simulink model "multirateEKFExample"  (R2018a)
settings: Solver=VariableStepAuto  StartTime=0.0  StopTime=t(end)  RelTol=1e-3
values from neighbouring files (symbols this model uses):
  Ts = 0.05    [MultirateNonlinearStateEstimationInSimulinkExample.m]
libraries: simulink x2, sharedTrackingLibrary x1
settings Model: Creator=The MathWorks, Inc.  LastModifiedBy=The MathWorks, Inc.
settings CodeAppCC: StateflowObjectComments=on

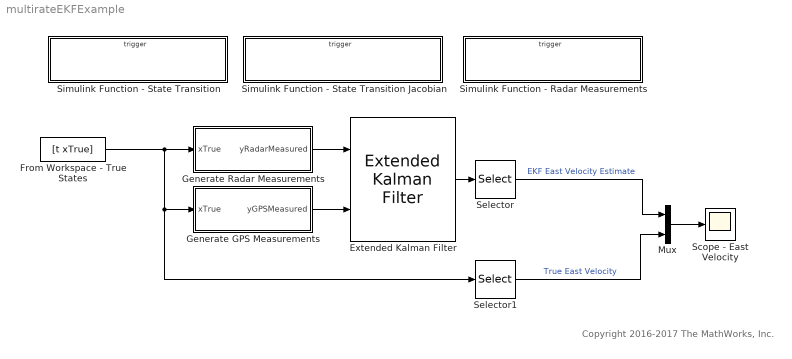
== system multirateEKFExample ==
  note: Copyright 2016-2017 The MathWorks, Inc.
  Extended Kalman Filter : sharedTrackingLibrary/Extended Kalman Filter  StateTransitionFcn=stateTransitionFcn  HasStateTransitionJacobianFcn=on  StateTransitionJacobianFcn=stateTransitionJacobianFcn  HasAdditiveProcessNoise=Nonadditive  ProcessNoise=[0.2 0; 0 0.2]  HasTimeVaryingProcessNoise=off  HasStateTransitionFcnExtraArgument=0  InitialState=[100; 100; 0; 0]  InitialStateCovariance=10  MeasurementFcn1=radarMeasurementFcn  HasMeasurementJacobianFcn1=off  HasMeasurementEnablePort1=off  HasAdditiveMeasurementNoise1=Nonadditive  MeasurementNoise1=[0.0025 0; 0 0.0025]  HasTimeVaryingMeasurementNoise1=off  HasMeasurementFcnExtraArgument1=0  MeasurementFcn2=gpsMeasurementFcn  HasMeasurementJacobianFcn2=off  HasMeasurementEnablePort2=off  HasAdditiveMeasurementNoise2=Additive  MeasurementNoise2=[100 0; 0 100]  HasTimeVaryingMeasurementNoise2=off  HasMeasurementFcnExtraArgument2=0  MeasurementFcn3=myMeasurementFcn  HasMeasurementJacobianFcn3=off  HasMeasurementEnablePort3=off  HasAdditiveMeasurementNoise3=Additive  MeasurementNoise3=1  HasTimeVaryingMeasurementNoise3=off  HasMeasurementFcnExtraArgument3=0  MeasurementFcn4=myMeasurementFcn  HasMeasurementJacobianFcn4=off  HasMeasurementEnablePort4=off  HasAdditiveMeasurementNoise4=Additive  MeasurementNoise4=1  HasTimeVaryingMeasurementNoise4=off  HasMeasurementFcnExtraArgument4=0  MeasurementFcn5=myMeasurementFcn  HasMeasurementJacobianFcn5=off  HasMeasurementEnablePort5=off  HasAdditiveMeasurementNoise5=Additive  MeasurementNoise5=1  HasTimeVaryingMeasurementNoise5=off  HasMeasurementFcnExtraArgument5=0  EnableMultirate=on  StateTransitionFcnSampleTime=0.05  MeasurementFcn1SampleTime=0.05  MeasurementFcn2SampleTime=1  MeasurementFcn3SampleTime=-1  MeasurementFcn4SampleTime=-1  MeasurementFcn5SampleTime=-1  UseCurrentEstimator=on  OutputStateCovariance=off  DataType=double  SampleTime=1  NumberOfMeasurements=2
      settings: SourceProductName=Control System Toolbox  SourceProductBaseCode=CT
  From Workspace - True States : FromWorkspace  VariableName=[t xTrue]  SampleTime=0
  Generate GPS Measurements : Subsystem
  Generate Radar Measurements : Subsystem
  Mux : Mux  Inputs=2
  Scope - East Velocity : Scope
  Selector : Selector  InputPortWidth=4  IndexOptions=Index vector (dialog)  Indices=3  OutputSizes=1
  Selector1 : Selector  InputPortWidth=4  IndexOptions=Index vector (dialog)  Indices=3  OutputSizes=1
  Simulink Function - Radar Measurements : Subsystem  TreatAsAtomicUnit=on
  Simulink Function - State Transition : Subsystem  TreatAsAtomicUnit=on
  Simulink Function - State Transition Jacobian : Subsystem  TreatAsAtomicUnit=on
  wires:
  From Workspace - True States/1 -> Selector1/1, Generate GPS Measurements/1(xTrue), Generate Radar Measurements/1(xTrue)
  Generate Radar Measurements/1(yRadarMeasured) -> Extended Kalman Filter/1
  Generate GPS Measurements/1(yGPSMeasured) -> Extended Kalman Filter/2
  Mux/1 -> Scope - East Velocity/1
  Selector1/1 -> Mux/2  "True East Velocity"
  Selector/1 -> Mux/1  "EKF East Velocity Estimate"
  Extended Kalman Filter/1 -> Selector/1

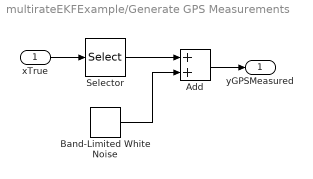
== system multirateEKFExample/Generate GPS Measurements ==
  xTrue : Inport  SampleTime=20*Ts
  Add : Sum
  Band-Limited White Noise : simulink/Sources/Band-Limited White Noise  Cov=50  Ts=20*Ts  seed=[23343;23344]
  Selector : Selector  InputPortWidth=4  IndexOptions=Index vector (dialog)  Indices=[1:2]  OutputSizes=1
  yGPSMeasured : Outport
  wires:
  xTrue/1 -> Selector/1
  Selector/1 -> Add/1
  Add/1 -> yGPSMeasured/1
  Band-Limited White Noise/1 -> Add/2

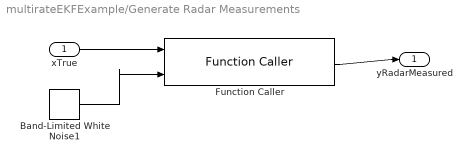
== system multirateEKFExample/Generate Radar Measurements ==
  xTrue : Inport  SampleTime=0.05
  Band-Limited White Noise1 : simulink/Sources/Band-Limited White Noise  Cov=5e-5  Ts=0.05  seed=[23341;23342]
  Function Caller : FunctionCaller  FunctionPrototype=y = radarMeasurementFcn(x,v)  InputArgumentSpecifications=zeros(4,1), zeros(2,1)  OutputArgumentSpecifications=zeros(2,1)
  yRadarMeasured : Outport
  wires:
  Function Caller/1 -> yRadarMeasured/1
  xTrue/1 -> Function Caller/1
  Band-Limited White Noise1/1 -> Function Caller/2

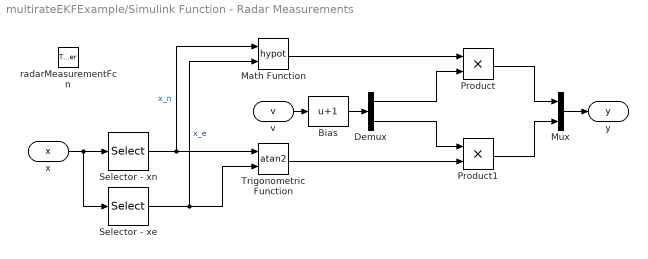
== system multirateEKFExample/Simulink Function - Radar Measurements ==
  radarMeasurementFcn : TriggerPort  TriggerType=function-call  IsSimulinkFunction=on  FunctionName=radarMeasurementFcn  VariantControl=Variant
  Bias : Bias  Bias=1
  Demux : Demux  Outputs=2
  Math Function : Math  Operator=hypot  SaturateOnIntegerOverflow=on
  Mux : Mux  Inputs=2
  Product : Product
  Product1 : Product
  Selector - xe : Selector  InputPortWidth=4  IndexOptions=Index vector (dialog)  Indices=1  OutputSizes=1
  Selector - xn : Selector  InputPortWidth=4  IndexOptions=Index vector (dialog)  Indices=2  OutputSizes=1
  Trigonometric Function : Trigonometry  Operator=atan2
  x : ArgIn  DisableCoverage=on  PortDimensions=4  ArgumentName=x
  v : ArgIn  DisableCoverage=on  Port=2  PortDimensions=2  ArgumentName=v
  y : ArgOut  DisableCoverage=on  PortDimensions=2  ArgumentName=y
  wires:
  Mux/1 -> y/1
  x/1 -> Selector - xe/1, Selector - xn/1
  Selector - xn/1 -> Math Function/1, Trigonometric Function/1  "x_n"
  Selector - xe/1 -> Math Function/2, Trigonometric Function/2  "x_e"
  Trigonometric Function/1 -> Product1/2
  v/1 -> Bias/1
  Math Function/1 -> Product/1
  Product/1 -> Mux/1
  Product1/1 -> Mux/2
  Bias/1 -> Demux/1
  Demux/1 -> Product/2
  Demux/2 -> Product1/1

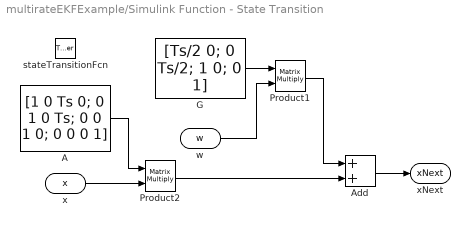
== system multirateEKFExample/Simulink Function - State Transition ==
  stateTransitionFcn : TriggerPort  TriggerType=function-call  IsSimulinkFunction=on  FunctionName=stateTransitionFcn  VariantControl=Variant
  A : Constant  Value=[1 0 Ts 0; 0 1 0 Ts; 0 0 1 0; 0 0 0 1]
  Add : Sum
  G : Constant  Value=[Ts/2 0; 0 Ts/2; 1 0; 0 1]
  Product1 : Product  Multiplication=Matrix(*)
  Product2 : Product  Multiplication=Matrix(*)
  x : ArgIn  DisableCoverage=on  PortDimensions=4  ArgumentName=x
  w : ArgIn  Port=2  PortDimensions=2  ArgumentName=w
  xNext : ArgOut  DisableCoverage=on  PortDimensions=4  ArgumentName=xNext
  wires:
  x/1 -> Product2/2
  A/1 -> Product2/1
  Product2/1 -> Add/2
  G/1 -> Product1/1
  w/1 -> Product1/2
  Product1/1 -> Add/1
  Add/1 -> xNext/1

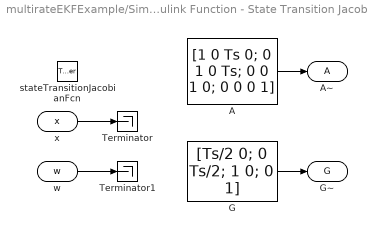
== system multirateEKFExample/Simulink Function - State Transition Jacobian ==
  stateTransitionJacobianFcn : TriggerPort  TriggerType=function-call  IsSimulinkFunction=on  FunctionName=stateTransitionJacobianFcn  VariantControl=Variant
  A : Constant  Value=[1 0 Ts 0; 0 1 0 Ts; 0 0 1 0; 0 0 0 1]
  G : Constant  Value=[Ts/2 0; 0 Ts/2; 1 0; 0 1]
  Terminator : Terminator
  Terminator1 : Terminator
  x : ArgIn  DisableCoverage=on  PortDimensions=4  ArgumentName=x
  w : ArgIn  Port=2  PortDimensions=2  ArgumentName=w
  A~ : ArgOut  DisableCoverage=on  PortDimensions=[4 4]  ArgumentName=A
  G~ : ArgOut  Port=2  PortDimensions=[4 2]  ArgumentName=G
  wires:
  G/1 -> G~/1
  x/1 -> Terminator/1
  w/1 -> Terminator1/1
  A/1 -> A~/1
